simulink model "ControladorTurbina"  (R2013b)
settings: Solver=ode3  StartTime=0.0  StopTime=80  FixedStep=0.002  RelTol=1e-3
InitFcn:
  | Alt = 2;
  | Vel =4;
  | wa = 72;
  | zetaA = 0.7;
  | load('../../Ganhos/BV9_30_03/GanhosTanqueHalf')
  | load('../../Dados_Input_Ganhos/BV9_30_03/sstanqueHalf_0')
  | [n,d] = butter(2,15*2*pi,'s')
  | F = tf(n,d);
  | Fd = c2d(F,0.01,'tustin');
  | [num, dem] = tfdata(Fd);
  | Ta = 100;
undefined symbols (not defined in the file or in its folder): dem, Kd, Kp, num, Plano_Long, sigbuilder_block
libraries: simulink x1
settings Model: Creator=AGSilva  LastModifiedBy=agsilva
settings DataIOCC: SignalLoggingSaveFormat=ModelDataLogs

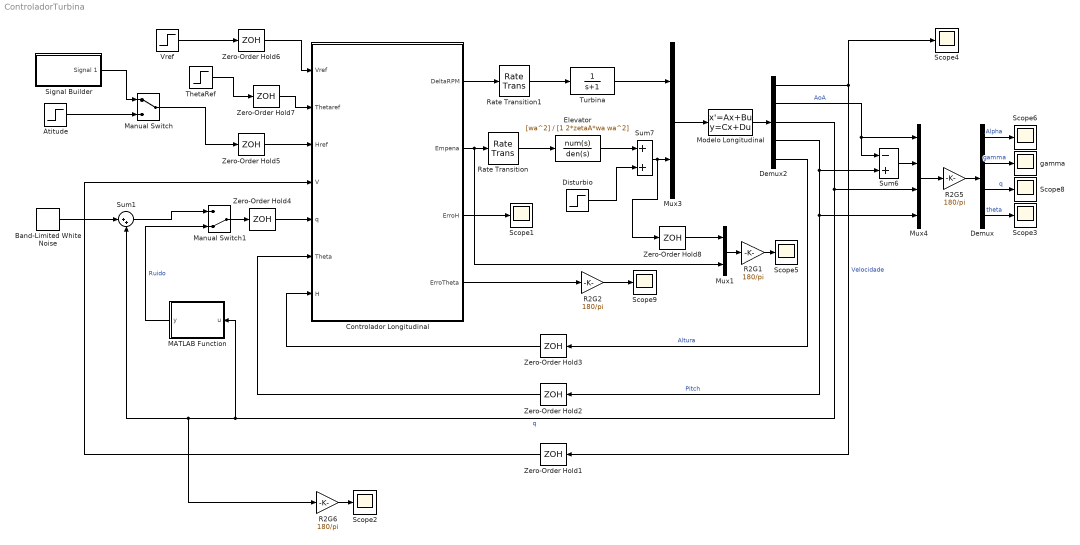
== system ControladorTurbina ==
  Atitude : Step  After=100*1  SampleTime=0
  Band-Limited White Noise : simulink/Sources/Band-Limited White Noise  Cov=0.004^2*0.002  Ts=0.002  seed=[23341]
  Controlador Longitudinal : Subsystem
  Demux : Demux
  Demux2 : Demux  Outputs=5
  Disturbio : Step  After=pi/180*0  SampleTime=0
  Elevator : TransferFcn  Numerator=[wa^2]  Denominator=[1 2*zetaA*wa wa^2]
  MATLAB Function : MATLAB Function  TreatAsAtomicUnit=on
  Manual Switch : ManualSwitch
  Manual Switch1 : ManualSwitch  CurrentSetting=0
  Modelo Longitudinal : StateSpace  A=Plano_Long(Alt,Vel).A  B=Plano_Long(Alt,Vel).B  C=eye(5)  D=zeros(5,2)  X0=[0 0 0 0 0]'
  Mux1 : Mux  Inputs=2
  Mux3 : Mux  Inputs=2
  Mux4 : Mux
  R2G{1..2,5..6} (4 alike) : Gain  Gain=180/pi
  Rate Transition : RateTransition
  Rate Transition1 : RateTransition
  Scope{1..6,8..9} (8 alike) : Scope
      Scope3 settings: SaveName=ScopeData3
      Scope4 settings: YMin=0.999999  YMax=1  SaveName=ScopeData2
      Scope5 settings: TimeRange=4.922600619195046  YMin=-0.06835511982570799  YMax=0.08720043572984756  SaveName=ScopeData4
      Scope6 settings: SaveName=ScopeData6
      Scope8 settings: SaveName=ScopeData8
      Scope9 settings: SaveName=ScopeData9
  Signal Builder : Subsystem  Tag=STV Subsys  LoadFcn=sigbuilder_block('load');  StartFcn=sigbuilder_block('start');  StopFcn=sigbuilder_block('stop');  ClipboardFcn=sigbuilder_block('clipboard');  mask(Sigbuilder block){}
      mask help: Simulink:masks:SigbuilderBlock_MD
      mask init:
      | if ~strcmp(get_param(bdroot(gcbh),'SimulationStatus'),'stopped') tuvar = sigbuilder_block('maskInit'); end
      settings: CopyFcn=sigbuilder_block('copy');  DeleteFcn=sigbuilder_block('delete');  ModelCloseFcn=sigbuilder_block('modelClose');  PreSaveFcn=sigbuilder_block('preSave');  PauseFcn=sigbuilder_block('pause');  ContinueFcn=sigbuilder_block('continue');  NameChangeFcn=sigbuilder_block('namechange');  OpenFcn=sigbuilder_block('open',[437.25 199.5 550.5 399.75 ]);  CloseFcn=sigbuilder_block('close');
      mask Display: plot(0, 0, 100, 100,[2, 2, 32, 32, 2], [68, 8, 8, 68, 68],[32, 2], [38, 38], [32, 19, 2],[53, 60, 44], [32, 17, 17, 2],[16, 16, 31, 31]);txt = getActiveGroup(gcbh);text(2, 100, txt,'verticalAlignment', 'top');
  Sum1 : Sum  Inputs=|++
  Sum6 : Sum  Inputs=-+
  Sum7 : Sum
  ThetaRef : Step  After=1*pi/180*1  SampleTime=0
  Turbina : TransferFcn  Denominator=[1 1]
  Vref : Step  After=10*0  SampleTime=0
  Zero-Order Hold{1..8} (8 alike) : ZeroOrderHold  SampleTime=1/Ta
  gamma : Scope
      settings: SaveName=ScopeData5
  wires:
  Modelo Longitudinal/1 -> Demux2/1
  Mux3/1 -> Modelo Longitudinal/1
  Demux2/2 -> Sum6/1, Mux4/1  "AoA"
  Demux/2 -> gamma/1  "gamma"
  Sum6/1 -> Mux4/2
  Demux2/1 -> Zero-Order Hold1/1, Scope4/1  "Velocidade"
  Turbina/1 -> Mux3/1
  Signal Builder/1(Signal 1) -> Manual Switch/1
  Atitude/1 -> Manual Switch/2
  Demux/1 -> Scope6/1  "Alpha"
  R2G6/1 -> Scope2/1
  Mux4/1 -> R2G5/1
  R2G5/1 -> Demux/1
  Demux/4 -> Scope3/1  "theta"
  Demux/3 -> Scope8/1  "q"
  Sum7/1 -> Zero-Order Hold8/1, Mux3/2
  R2G2/1 -> Scope9/1
  Manual Switch/1 -> Zero-Order Hold5/1
  Elevator/1 -> Sum7/1
  Disturbio/1 -> Sum7/2
  Vref/1 -> Zero-Order Hold6/1
  Demux2/5 -> Zero-Order Hold3/1  "Altura"
  Demux2/4 -> Sum6/2, Mux4/4, Zero-Order Hold2/1  "Pitch"
  Band-Limited White Noise/1 -> Sum1/1
  Demux2/3 -> Mux4/3, R2G6/1, Sum1/2, MATLAB Function/1(u)  "q"
  Controlador Longitudinal/4(ErroTheta) -> R2G2/1
  Controlador Longitudinal/3(ErroH) -> Scope1/1
  Zero-Order Hold1/1 -> Controlador Longitudinal/4(V)
  Zero-Order Hold2/1 -> Controlador Longitudinal/6(Theta)
  Zero-Order Hold3/1 -> Controlador Longitudinal/7(H)
  Zero-Order Hold4/1 -> Controlador Longitudinal/5(q)
  Zero-Order Hold5/1 -> Controlador Longitudinal/3(Href)
  Zero-Order Hold6/1 -> Controlador Longitudinal/1(Vref)
  Zero-Order Hold7/1 -> Controlador Longitudinal/2(Thetaref)
  ThetaRef/1 -> Zero-Order Hold7/1
  Rate Transition/1 -> Elevator/1
  Rate Transition1/1 -> Turbina/1
  Controlador Longitudinal/2(Empena) -> Mux1/2, Rate Transition/1
  Controlador Longitudinal/1(DeltaRPM) -> Rate Transition1/1
  R2G1/1 -> Scope5/1
  Mux1/1 -> R2G1/1
  Zero-Order Hold8/1 -> Mux1/1
  Manual Switch1/1 -> Zero-Order Hold4/1
  Sum1/1 -> Manual Switch1/1
  MATLAB Function/1(y) -> Manual Switch1/2  "Ruido"

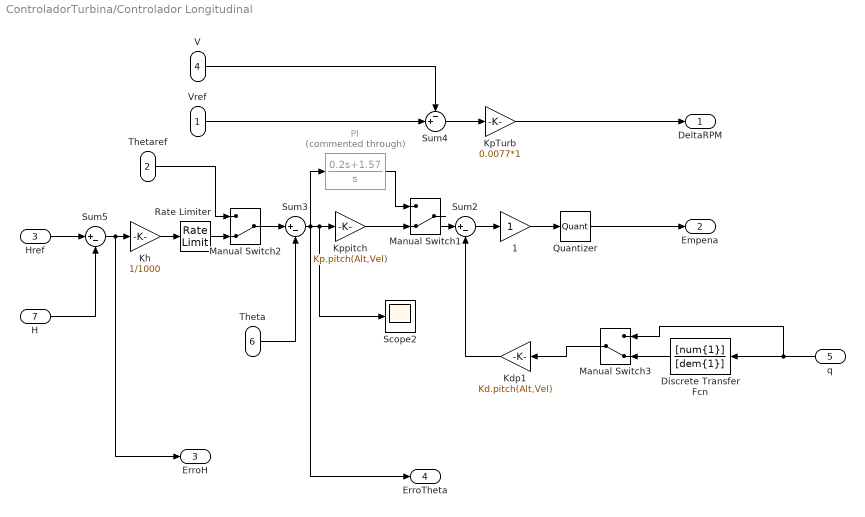
== system ControladorTurbina/Controlador Longitudinal ==
  Vref : Inport
  Thetaref : Inport  Port=2
  Href : Inport  Port=3
  V : Inport  Port=4
  q : Inport  Port=5
  Theta : Inport  Port=6
  H : Inport  Port=7
  1 : Gain
  Discrete Transfer Fcn : DiscreteTransferFcn  Numerator=[num{1}]  Denominator=[dem{1}]
  Kdp1 : Gain  Gain=Kd.pitch(Alt,Vel)
  Kh : Gain  Gain=1/1000
  KpTurb : Gain  Gain=0.0077*1
  Kppitch : Gain  Gain=Kp.pitch(Alt,Vel)
  Manual Switch1 : ManualSwitch  CurrentSetting=0
  Manual Switch2 : ManualSwitch  CurrentSetting=0
  Manual Switch3 : ManualSwitch  CurrentSetting=0
  PI : TransferFcn  Commented=through  Numerator=[0.2 1.57]  Denominator=[1 0]
  Quantizer : Quantizer  QuantizationInterval=0.005*pi/180
  Rate Limiter : RateLimiter  RisingSlewLimit=1*pi/180  FallingSlewLimit=-1*pi/180  SampleTimeMode=inherited
  Scope2 : Scope
      settings: SaveName=ScopeData7
  Sum2 : Sum  Inputs=|+-
  Sum3 : Sum  Inputs=|+-
  Sum4 : Sum  Inputs=-+|
  Sum5 : Sum  Inputs=|+-
  DeltaRPM : Outport
  Empena : Outport  Port=2
  ErroH : Outport  Port=3
  ErroTheta : Outport  Port=4
  wires:
  Sum3/1 -> ErroTheta/1, Scope2/1, Kppitch/1, PI/1
  Kdp1/1 -> Sum2/2
  Sum4/1 -> KpTurb/1
  Sum5/1 -> ErroH/1, Kh/1
  KpTurb/1 -> DeltaRPM/1
  Href/1 -> Sum5/1
  Manual Switch1/1 -> Sum2/1
  Kppitch/1 -> Manual Switch1/2
  PI/1 -> Manual Switch1/1
  Manual Switch2/1 -> Sum3/1
  Kh/1 -> Rate Limiter/1
  Sum2/1 -> 1/1
  1/1 -> Quantizer/1
  q/1 -> Discrete Transfer Fcn/1, Manual Switch3/1
  Discrete Transfer Fcn/1 -> Manual Switch3/2
  Manual Switch3/1 -> Kdp1/1
  Rate Limiter/1 -> Manual Switch2/2
  Vref/1 -> Sum4/2
  V/1 -> Sum4/1
  Thetaref/1 -> Manual Switch2/1
  Theta/1 -> Sum3/2
  H/1 -> Sum5/2
  Quantizer/1 -> Empena/1

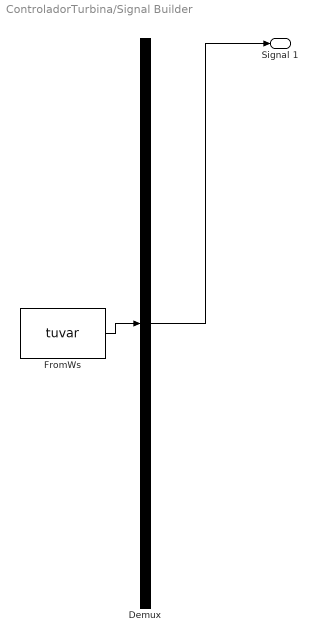
== system ControladorTurbina/Signal Builder ==
  Demux : Demux  Tag=STV Demux  Outputs=1
  FromWs : FromWorkspace  Tag=STV FromWs  VariableName=tuvar  SampleTime=0
      SigBuilderData=|
      | common.afterFinalStr = 'Extrapolate'
      | common.sampleTime = 0
      | dataSet.timeRange = [0 80]
      | dataSet.name = 'Group 1'
      | sbobj.Groups.Name = 'Group 1'
      | sbobj.Groups.Signals.Name = 'Signal 1'
      | sbobj.Groups.Signals.XData = [0 5 30 50 70 80]
      | sbobj.Groups.Signals.YData = [0 1 250 250 0 0]
      | sbobj.Groups.TimeRange = [0 80]
  Signal 1 : Outport  Tag=STV Outport
  wires:
  Demux/1 -> Signal 1/1
  FromWs/1 -> Demux/1

== matlab function ControladorTurbina/MATLAB Function ==
  data: u input; y output
function y = fcn(u)
%#codegen
desviop = 0.004;

y = u + desviop*randn(1,1);
